simulink model "psbdcdrive_disc"  (Simulink 6.0)
settings: Solver=FixedStepDiscrete  SolverMode=SingleTasking  StartTime=0.0  StopTime=2  FixedStep=Ts  RelTol=1e-3  AbsTol=1e-3
PreLoadFcn:
  | assignin('base','Ts',[10e-6])
InitFcn:
  | powericon('psbinitsys',bdroot);
undefined symbols (not defined in the file or in its folder): Ts
libraries: powerlib2 x10, powerlib_extras x2
settings Model: Creator=patrice  LastModifiedBy=batserve  ExtModeTrigMode=oneshot  ExtModeArmWhenConnect=off  ExtModeAutoUpdateStatusClock=off
settings DataIOCC: LimitDataPoints=off  SaveFinalState=on  SaveFormat=StructureWithTime  SaveOutput=off  SaveTime=off  SignalLoggingName=sigsOut
settings OptimizationCC: BlockReduction=off  BooleanDataType=off
settings DebuggingCC: CheckExecutionContextPreStartOutputMsg=on  CheckExecutionContextRuntimeOutputMsg=on  SolverPrmCheckMsg=none  UnconnectedInputMsg=none  UnconnectedOutputMsg=none
settings HardwareCC: TargetUnknown=on
settings RTWCC: TemplateMakefile=grt_unix.tmf

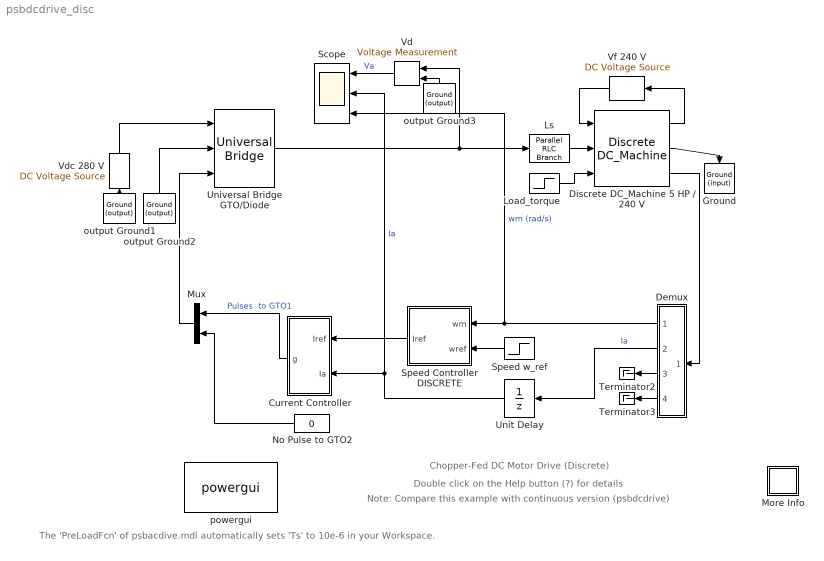
== system psbdcdrive_disc ==
  note: Chopper-Fed DC Motor Drive (Discrete)
  note: Double click on the Help button (?) for details
  note: Note: Compare this example with continuous version (psbdcdrive)
  note: The 'PreLoadFcn' of psbacdive.mdl
      | automatically sets 'Ts' to 10e-6 in your Workspace.
  Current Controller : Subsystem  Orientation=left  mask{h=2}
      mask prompts: h "Hysteresis band (A)"
      mask help: Hysteresis Current Controller
      mask Display: plot(0,0,100,100,[45,45],[35,65],[55,55],[35,65],[45,65],[65,65],[35,55],[35,35])
  Demux : Subsystem  Orientation=left
  Discrete DC_Machine 5 HP / 240 V : powerlib_extras/Additional Machines/Discrete DC_Machine  RLa="[0.5  0.01]"  RLf="[240  0]"  Laf=1.23  J=0.05  Bm=0.02  Tf=0  w0=0  PSBOutputType=110  Ts=Ts
  Ground : powerlib2/Connectors/Ground (input)  Tag=PoWeRsYsTeMbLoCk  Orientation=down
  "Load_torque " : Step  Time=1.5  Before=5  After=25  SampleTime=0
  Ls : powerlib2/Elements/Parallel RLC Branch  Tag=PoWeRsYsTeMbLoCk  a=inf  b=10e-03  c=0  mesure=None  PSBOutputType=1
  More Info : Subsystem
      mask Display: disp('?')
  Mux : Mux  Orientation=left  Inputs=2
  No Pulse to GTO2 : Constant  Orientation=left  Value=0
  Scope : Scope  NumInputPorts=3
      settings: TickLabels=on  YMin=-100~0~-25  YMax=300~35~150  SaveName=var
  Speed Controller DISCRETE : Subsystem  Orientation=left  mask(PI controller){Kp=1.6, Ki=16, Ilim=30, Ts=Ts}
      mask prompts: Kp "Proportional gain (Kp)"; Ki "Integral gain (Ki)"; Ilim "Current limit (A)"; Ts "Sample time (s) :"
      mask help: Proportional-Integral Speed Controller
      mask Display: plot(0,0,100,100,[35,35,65],[70,30,30],[35,65],[45,60])
  "Speed w_ref " : Step  Orientation=left  Time=0.8  Before=120  After=160  SampleTime=0
  Terminator2 : Terminator
  Terminator3 : Terminator
  Unit Delay : UnitDelay  Orientation=left  SampleTime=Ts
  Universal Bridge GTO/Diode : powerlib2/Power Electronics/Universal Bridge  Tag=PoWeRsYsTeMbLoCk  arms=1  confi=ABC as output terminals  injcc=10000  cf=inf  device=GTO / Diodes  Ron=0.05  Lon=0  VFs="[  1  1  ]"  Vf=.8  gtoparameters=[ 10e-6 , 20e-6 ]  igbtparameters=[ 1e-6 , 2e-6 ]  mesure=None  PSBOutputType=111
  Vd : powerlib2/Measurements/Voltage Measurement  Tag=PoWeRsYsTeMmEaSuReMeNt  Orientation=left  PhasorSimulation=off  OutputType=Magnitude  PSBOutputType=0  PSBequivalent=0
  "Vdc 280 V " : powerlib2/Electrical Sources/DC Voltage Source  Tag=PoWeRsYsTeMbLoCk  Orientation=up  V=280  mesure=None  PSBOutputType=1
  Vf 240 V : powerlib2/Electrical Sources/DC Voltage Source  Tag=PoWeRsYsTeMbLoCk  Orientation=left  V=240  mesure=None  PSBOutputType=1
  output Ground1 : powerlib2/Connectors/Ground (output)  Tag=PoWeRsYsTeMbLoCk  Orientation=up  PSBOutputType=1
  output Ground2 : powerlib2/Connectors/Ground (output)  Tag=PoWeRsYsTeMbLoCk  Orientation=up  PSBOutputType=1
  output Ground3 : powerlib2/Connectors/Ground (output)  Tag=PoWeRsYsTeMbLoCk  Orientation=up  PSBOutputType=1
  powergui : powerlib2/powergui  Frange=[0:2:500]  Ylog=off  Xlog=on  save=off  variable=ZData  ZoomFFT=on  StartTime=0.0  cycles=1  DisplayStyle=off  fundamental=60  FreqAxis=off  MaxFrequency=1000  frequencyindice=1  frequencyindicesteady=1  RmsSteady=1  display=off  Ts=10e-6  methode=off  frequency=60  echomessages=off
  wires:
  "Vdc 280 V "/1 -> Universal Bridge GTO/Diode/1
  output Ground1/1 -> "Vdc 280 V "/1
  Ls/1 -> Discrete DC_Machine 5 HP / 240 V/2
  Vf 240 V/1 -> Discrete DC_Machine 5 HP / 240 V/1
  Speed Controller DISCRETE/1(Iref) -> Current Controller/1(Iref)
  Unit Delay/1 -> Current Controller/2(Ia), Scope/2  "Ia"
  Discrete DC_Machine 5 HP / 240 V/2 -> Ground/1
  Discrete DC_Machine 5 HP / 240 V/1 -> Vf 240 V/1
  Discrete DC_Machine 5 HP / 240 V/3 -> Demux/1(m)
  Demux/1(wm) -> Speed Controller DISCRETE/1(wm), Scope/3  "wm (rad/s)"
  Demux/2(Ia) -> Unit Delay/1  "Ia"
  Demux/4(Te) -> Terminator3/1
  Demux/3(If) -> Terminator2/1
  Current Controller/1(g) -> Mux/1  "Pulses  to GTO1"
  Mux/1 -> Universal Bridge GTO/Diode/3
  output Ground2/1 -> Universal Bridge GTO/Diode/2
  Universal Bridge GTO/Diode/1 -> Ls/1, Vd/1
  "Speed w_ref "/1 -> Speed Controller DISCRETE/2(wref)
  "Load_torque "/1 -> Discrete DC_Machine 5 HP / 240 V/3
  No Pulse to GTO2/1 -> Mux/2
  Vd/1 -> Scope/1  "Va"
  output Ground3/1 -> Vd/2

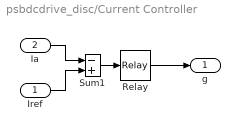
== system psbdcdrive_disc/Current Controller ==
  Iref : Inport  Port=1  LatchInput=off
  Ia : Inport  Port=2  LatchInput=off
  Relay : Relay  OnSwitchValue=h/2  OffSwitchValue=-h/2
  Sum1 : Sum  Inputs=-+  SaturateOnIntegerOverflow=on  InputSameDT=on
  g : Outport  InitialOutput=0
  wires:
  Sum1/1 -> Relay/1
  Relay/1 -> g/1
  Ia/1 -> Sum1/1
  Iref/1 -> Sum1/2

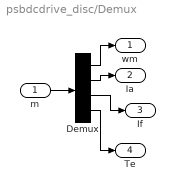
== system psbdcdrive_disc/Demux ==
  m : Inport  Port=1  LatchInput=off
  Demux : Demux
  wm : Outport
  Ia : Outport  Port=2
  If : Outport  Port=3
  Te : Outport  Port=4
  wires:
  Demux/1 -> wm/1
  Demux/2 -> Ia/1
  m/1 -> Demux/1
  Demux/3 -> If/1
  Demux/4 -> Te/1

== system psbdcdrive_disc/More Info ==
  note: Chopper-Fed DC Motor Drive (Discrete)
  note: Circuit Description
  note: Demonstration
  note: A DC motor is fed by a DC source through a chopper which consists of GTO thyristor and a free-wheeling diode.
      |
      | The  GTO and diode are simulated with the Universal Bridge block where the number of arms has been set to 1
      | and the  specified power electronic device  is  GTO/Diode. Each switch on the block icon represents a GTO/antiparallel diode pair.
      | Pulses are sent to the top GTO1  only. No pulses are sent to the bottom GTO2.
      | Therefore Diode2 will act as a free wheeling diode.
      |
      | The advantage of using the Universal Bridge block is that  it can be discretized and allows faster simultion speeds
      | than with an individual GTO and Diode. Also, when a purely resistive snubber is used
      | the commutation from GTO to Diode is instantaneous and cleaner wavehapes is obtained for voltage Va
      |
      | The motor drives a mechanical load characterized by inertia J, friction coeficient B, and load torque TL.
      | The motor uses the discrete DC machine provided in the Extras/Additional Machines library.
      |
      | The hysteresis current controller compares the sensed current with the reference and generates
      | the trigger signal for the GTO thyristor to force the motor current to follow the reference.
      | The speed control loop uses a proportional-integral controller which produces the reference for the current loop.
      | Current and Voltage Measurement blocks provide signals for visualization purpose.
  note: Start the simulation and observe the motor voltage (Va), current (Ia) and speed  (wm) on the scope.
      | The following observations can be made:
  note: 0< t < 0.8 s: Starting and Steady State Operation
  note: The reference speed  is increased from 120 rad/s to 160 rad/s.
      | The speed controller regulates the speed in approximately 0.25 s and the average current stabilizes at 6.6 A.
      | During the transient period, current is still maintained at 30 A.
  note: During this period, the load torque is TL = 5.N.m and the motor reaches the reference speed (wref = 120 rad/s) given to the speed controller .
      | The initial values of reference torque and speed are set in the two Step blocks connected to the TL torque input of the motor.
      | Notice that during the motor starting the current is maintained to 30 A, according to the current limit set in the speed regulator.
      | Zoom in the motor current Ia in steady state. Observe the current triangular waveshape varying between 5 A and 7 A,
      | corresponding to the specified hysteresis of 2 A. The commutation frequency is approximately 1.5 kHz.
  note: H. LeHuy (Universite Laval, Quebec) and G. Sybille (Hydro-Quebec)
  note: t = 0.8 s : Reference Speed Step
  note: t = 1.5 s : Load Torque Step
  note: The load torque is suddenly  increased from  5 N.m to  25 N.m.
      | The current increases to 23 A, while the speed is maintained at the 160 rad/s set point.
  note: Note: This example is similar to the continuous version also provided in the Demos library, but discretisation allows faster simulation.

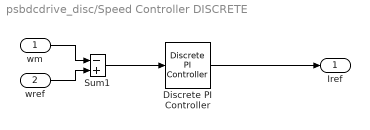
== system psbdcdrive_disc/Speed Controller DISCRETE ==
  wm : Inport  Port=1  LatchInput=off
  wref : Inport  Port=2  LatchInput=off
  Discrete PI Controller : powerlib_extras/Discrete  Control Blocks/Discrete PI Controller  Kp=Kp  Ki=Ki  Par_Limits=[Ilim -Ilim]  Init=0  Ts=Ts
  Sum1 : Sum  Inputs=-+  SaturateOnIntegerOverflow=on  InputSameDT=on
  Iref : Outport  InitialOutput=0
  wires:
  wref/1 -> Sum1/2
  wm/1 -> Sum1/1
  Sum1/1 -> Discrete PI Controller/1
  Discrete PI Controller/1 -> Iref/1
